simulink model "Project3Simulink"  (R2020a)
settings: Solver=VariableStepAuto  StartTime=0.0  StopTime=10.0  RelTol=1e-3
values from neighbouring files (symbols this model uses):
  A = 3    [Project3.m]
  F = 2    [Project3.m]
  Ti = 5    [Project3.m]
settings Model: Creator=cresp  LastModifiedBy=cresp

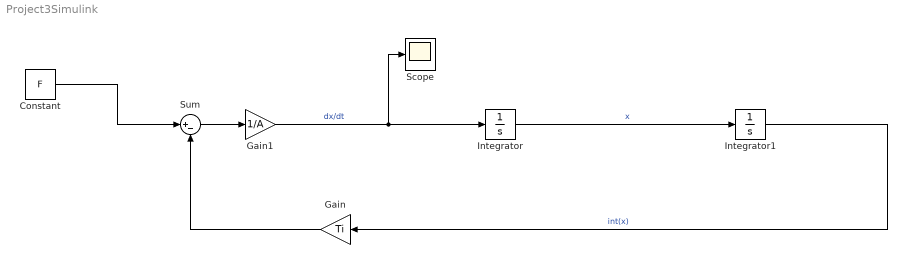
== system Project3Simulink ==
  Constant : Constant  Value=F
  Gain : Gain  Gain=Ti
  Gain1 : Gain  Gain=1/A
  Integrator : Integrator
  Integrator1 : Integrator
  Scope : Scope
  Sum : Sum  Inputs=|+-
  wires:
  Gain1/1 -> Scope/1, Integrator/1  "dx/dt"
  Integrator/1 -> Integrator1/1  "x"
  Integrator1/1 -> Gain/1  "int(x)"
  Gain/1 -> Sum/2
  Constant/1 -> Sum/1
  Sum/1 -> Gain1/1
